simulink model "SIMULAZIONE_gruppoE"  (R2020b)
settings: Solver=VariableStepAuto  StartTime=0.0  StopTime=10.0  RelTol=1e-3
model workspace (MAT data in the model file):
  s = Simulink.Parameter
  s.DataType = 'auto'
  s.Dimensions = [0 0]
values from neighbouring files (symbols this model uses):
  A = [0,1; -981/1550, -80/31]    [PROGETTO_gruppoE.m]
  B = [0;40/31]    [PROGETTO_gruppoE.m]
  C = [0,1]    [PROGETTO_gruppoE.m]
  den_r = d_r{1}    [PROGETTO_gruppoE.m]
  num_r = n_r{1}    [PROGETTO_gruppoE.m]
  omega_n = 100    [PROGETTO_gruppoE.m]
  W = 5    [PROGETTO_gruppoE.m]
  x0 = [0;0]    [PROGETTO_gruppoE.m]
settings Model: Creator=super  LastModifiedBy=probook

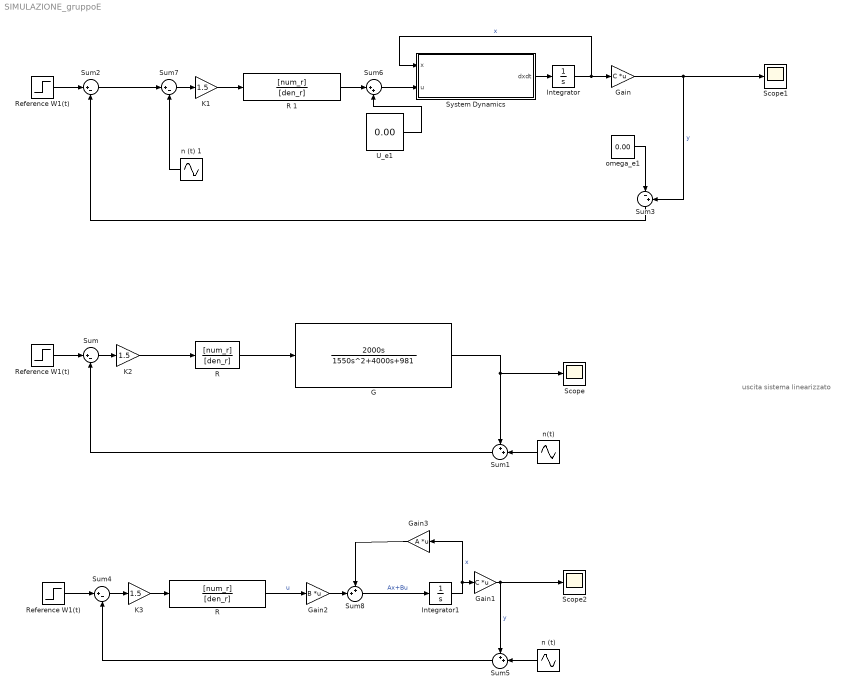
== system SIMULAZIONE_gruppoE ==
  note: uscita sistema linearizzato
  G : TransferFcn  Numerator=[2000,0]  Denominator="[1550,  4000, 981]"
  Gain : Gain  Gain=C  Multiplication=Matrix(K*u)
  Gain1 : Gain  Gain=C  Multiplication=Matrix(K*u)
  Gain2 : Gain  Gain=B  Multiplication=Matrix(K*u)
  Gain3 : Gain  Gain=A  Multiplication=Matrix(K*u)
  Integrator : Integrator  InitialCondition=x0
  Integrator1 : Integrator  InitialCondition=x0
  K1 : Gain  Gain=1.5
  K2 : Gain  Gain=1.5
  K3 : Gain  Gain=1.5
  R : TransferFcn  Numerator=[num_r]  Denominator=[den_r]
  "R " : TransferFcn  Numerator=[num_r]  Denominator=[den_r]
  R 1 : TransferFcn  Numerator=[num_r]  Denominator=[den_r]
  Reference W1(t) : Step  After=W  SampleTime=0
  "Reference W1(t) " : Step  After=W  SampleTime=0
  "Reference W1(t) " : Step  After=W  SampleTime=0
  Scope : Scope
  Scope1 : Scope
  Scope2 : Scope
  Sum{,2,4,7} (4 alike) : Sum  Inputs=|+-
  Sum1 : Sum  Inputs=++|
  Sum3 : Sum  Inputs=|-+
  Sum5 : Sum  Inputs=++|
  Sum6 : Sum  Inputs=|++
  Sum8 : Sum  Inputs=++|
  System Dynamics : MATLAB Function  TreatAsAtomicUnit=on
  U_e1 : Constant  Value=0.00
  "n (t) " : Sin  Amplitude=0.02  Frequency=omega_n  SampleTime=0
  n (t) 1 : Sin  Amplitude=0.02  Frequency=omega_n  SampleTime=0
  n(t) : Sin  Amplitude=0.02  Frequency=omega_n  SampleTime=0
  omega_e1 : Constant  Value=0.00
  wires:
  System Dynamics/1(dxdt) -> Integrator/1
  Gain/1 -> Sum3/2, Scope1/1  "y"
  Integrator/1 -> System Dynamics/1(x), Gain/1  "x"
  "Reference W1(t) "/1 -> Sum2/1
  R 1/1 -> Sum6/1
  Sum2/1 -> Sum7/1
  Sum3/1 -> Sum2/2
  Sum6/1 -> System Dynamics/2(u)
  U_e1/1 -> Sum6/2
  Sum7/1 -> K1/1
  n (t) 1/1 -> Sum7/2
  K1/1 -> R 1/1
  omega_e1/1 -> Sum3/1
  "n (t) "/1 -> Sum5/2
  Gain3/1 -> Sum8/1
  Gain2/1 -> Sum8/2
  "R "/1 -> Gain2/1  "u"
  Sum4/1 -> K3/1
  Gain1/1 -> Sum5/1, Scope2/1  "y"
  Sum5/1 -> Sum4/2
  Sum8/1 -> Integrator1/1  "Ax+Bu"
  G/1 -> Scope/1, Sum1/1
  Sum1/1 -> Sum/2
  Integrator1/1 -> Gain1/1, Gain3/1  "x"
  R/1 -> G/1
  Reference W1(t)/1 -> Sum/1
  Sum/1 -> K2/1
  "Reference W1(t) "/1 -> Sum4/1
  n(t)/1 -> Sum1/2
  K2/1 -> R/1
  K3/1 -> "R "/1

== matlab function SIMULAZIONE_gruppoE/System Dynamics ==
  data: x input; u input; dxdt output
function dxdt  = systemDynamic(x,u)
beta = 2;
massa = 0.1;
e_i = 0.5;
inerzia = 0.75; %Ie
gg=9.81;

dx1dt=x(2);  %x1=theta
dx2dt=(-beta*x(2)-gg*massa*e_i*sin(x(1))+u)/(massa*e_i*e_i+inerzia);  %x2=omega
%dxdt = [dx1dt; dx2dt; dx3dt;...;dxndt];
dxdt = [dx1dt; dx2dt;];
